simulink model "Edge_Detector"  (R2025b)
settings: Solver=FixedStepDiscrete  StartTime=0.0  StopTime=10.0  FixedStep=0.01  RelTol=1e-3
libraries: simulink x3
settings Model: Creator=soura  LastModifiedBy=soura

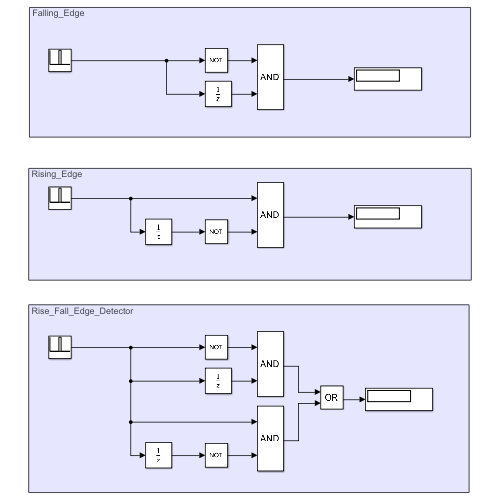
[thumbnail: Simulink's stored preview of the top-level diagram]
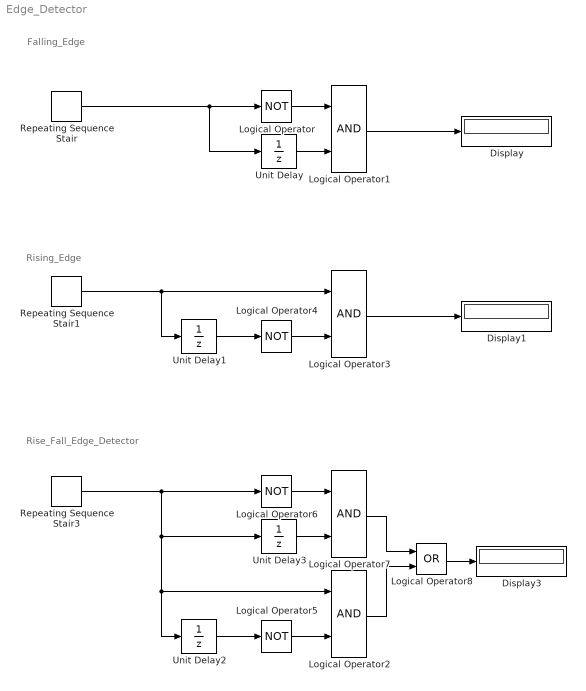
== system Edge_Detector ==
  note: Rise_Fall_Edge_Detector
  note: Rising_Edge
  note: Falling_Edge
  Display : Display
  Display1 : Display
  Display3 : Display
  Logical Operator{,4..6} (4 alike) : Logic  Operator=NOT  AllPortsSameDT=off  OutDataTypeStr=boolean
  Logical Operator{1..3,7} (4 alike) : Logic  AllPortsSameDT=off  OutDataTypeStr=boolean
  Logical Operator8 : Logic  Operator=OR  AllPortsSameDT=off  OutDataTypeStr=boolean
  Repeating Sequence Stair : simulink/Sources/Repeating Sequence Stair  OutValues=[0 0 0 1 0 0 0].'  tsamp=-1  OutMin=[]  OutMax=[]  OutDataTypeStr=double  OutputDataTypeScalingMode=double  OutDataType=fixdt(0,8)  ConRadixGroup=Best Precision: Vector-wise  OutScaling=2^-12
  Repeating Sequence Stair1 : simulink/Sources/Repeating Sequence Stair  OutValues=[0 0 0 1 0 0 0].'  tsamp=-1  OutMin=[]  OutMax=[]  OutDataTypeStr=double  OutputDataTypeScalingMode=double  OutDataType=fixdt(0,8)  ConRadixGroup=Best Precision: Vector-wise  OutScaling=2^-12
  Repeating Sequence Stair3 : simulink/Sources/Repeating Sequence Stair  OutValues=[0 0 0 1 0 0 0].'  tsamp=-1  OutMin=[]  OutMax=[]  OutDataTypeStr=double  OutputDataTypeScalingMode=double  OutDataType=fixdt(0,8)  ConRadixGroup=Best Precision: Vector-wise  OutScaling=2^-12
  Unit Delay{,1..3} (4 alike) : UnitDelay  SampleTime=-1  HasFrameUpgradeWarning=on
  wires:
  Logical Operator/1 -> Logical Operator1/1
  Unit Delay/1 -> Logical Operator1/2
  Repeating Sequence Stair/1 -> Unit Delay/1, Logical Operator/1
  Logical Operator1/1 -> Display/1
  Logical Operator3/1 -> Display1/1
  Repeating Sequence Stair1/1 -> Logical Operator3/1, Unit Delay1/1
  Unit Delay1/1 -> Logical Operator4/1
  Logical Operator4/1 -> Logical Operator3/2
  Repeating Sequence Stair3/1 -> Unit Delay3/1, Logical Operator2/1, Unit Delay2/1, Logical Operator6/1
  Unit Delay2/1 -> Logical Operator5/1
  Logical Operator5/1 -> Logical Operator2/2
  Logical Operator6/1 -> Logical Operator7/1
  Unit Delay3/1 -> Logical Operator7/2
  Logical Operator7/1 -> Logical Operator8/1
  Logical Operator2/1 -> Logical Operator8/2
  Logical Operator8/1 -> Display3/1
